simulink model "moto_linearization"  (R2026a)
settings: Solver=VariableStepAuto  StopTime=30
values from neighbouring files (symbols this model uses):
  ft = bs.FrontTire    [bikeSimToMotoParameters.m]
  Gf = Nsh.'*(Oh - B)    [bikeSimToMotoParameters.m]
  Ib = sum(I,3)    [bikeSimToMotoParameters.m]
  If = sum(I,3)    [bikeSimToMotoParameters.m]
  Ift = zeros(3)    [bikeSimToMotoParameters.m]
  Irt = zeros(3)    [bikeSimToMotoParameters.m]
  m = front_bodies(k).m    [bikeSimToMotoParameters.m]
  N = eye(3)    [bikeSimToMotoParameters.m]
  Ob = sum([rear_bodies.O].*[rear_bodies.m],2)/p.mb    [bikeSimToMotoParameters.m]
  p = motoParameters    [bikeSimToMotoParameters.m]    (also in moto_init.m = bikeSimToPrydeV2Parameters(bs,130/3.6); moto_trim_test.m = P{idx_vx}; steadyTurningTrimEqns.m = in3(41,:); steadyTurningTrimJac.m = in3(41,:))
  pf = fpacejka(bs.FrontTire.Pacejka)    [moto_trim_test.m]
  pr = fpacejka(bs.RearTire.Pacejka)    [moto_trim_test.m]
  rt = bs.RearTire    [bikeSimToMotoParameters.m]
  s = linspace(-pi,pi,36)'    [moto_init.m]
  sm = bs.SprungMass    [bikeSimToMotoParameters.m]
  X = zeros(ns,ns,12)    [moto_trim_test.m]
undefined symbols (not defined in the file or in its folder): mb, mh, Rr, Vlow, Y, Z
libraries: sm_lib x60, nesl_utility x51
(part 3 of 5)

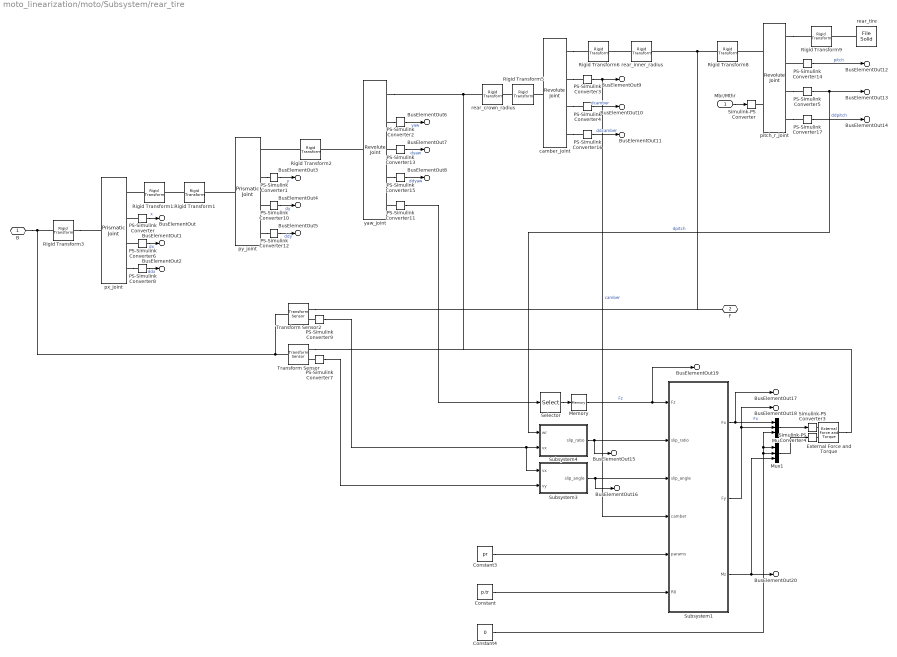
== system moto_linearization/moto/Subsystem/rear_tire ==
  Mbr/Mthr : Inport
  Constant : Constant  Value=p.tr
  Constant3 : Constant  Value=pr
  Constant4 : Constant  Value=0
  External Force and Torque : sm_lib/Forces and Torques/External Force and Torque  EnableForceX=off  EnableForceY=off  EnableForceZ=off  EnableForce=on  ForceResolutionFrame=AttachedFrame  EnableTorqueX=off  EnableTorqueY=off  EnableTorqueZ=off  EnableTorque=on  TorqueResolutionFrame=AttachedFrame
  Memory : Memory  InitialCondition=p.fzr  LinearizeAsDelay=on
  Mux : Mux  Inputs=3
  Mux1 : Mux  Inputs=3
  PS-Simulink Converter{,1..17} (18 alike) : nesl_utility/PS-Simulink Converter  PhysicalDomain=network_engine_domain  SubClassName=ps_output  LeftPortType=input  RightPortType=output  PseudoPeriodic=off  Frequencies=[]  VectorFormat=inherit  Unit=inherit  AffineConversion=off
  Rigid Transform1 : sm_lib/Frames and Transforms/Rigid Transform  RotationMethod=StandardAxis  FollAlignAxisA=+X  BaseAlignAxisA=+Y  FollAlignAxisB=+Y  BaseAlignAxisB=+Z  RotationStandardAxis=-X  RotationAngle=90  RotationAngleUnits=deg  RotationArbitraryAxis=[0 0 1]  RotationSequenceAxes=FollowerAxes  RotationSequence=XYX  RotationSequenceAngles=[0 0 0]  RotationSequenceAnglesUnits=deg  RotationMatrix=[1 0 0;0 1 0;0 0 1]  Quaternion=[1 0 0 0]  TranslationMethod=None  TranslationCartesianOffset=[0 0 0]  TranslationCartesianOffsetUnits=m  TranslationStandardAxis=+Z  TranslationStandardOffset=0  TranslationStandardOffsetUnits=m  TranslationROffset=0  TranslationROffsetUnits=m  TranslationThetaOffset=0  TranslationThetaOffsetUnits=deg  TranslationZOffset=0  TranslationZOffsetUnits=m
  Rigid Transform12 : sm_lib/Frames and Transforms/Rigid Transform  RotationMethod=StandardAxis  FollAlignAxisA=+X  BaseAlignAxisA=+Y  FollAlignAxisB=+Y  BaseAlignAxisB=+Z  RotationStandardAxis=-Y  RotationAngle=90  RotationAngleUnits=deg  RotationArbitraryAxis=[0 0 1]  RotationSequenceAxes=FollowerAxes  RotationSequence=XYX  RotationSequenceAngles=[0 0 0]  RotationSequenceAnglesUnits=deg  RotationMatrix=[1 0 0;0 1 0;0 0 1]  Quaternion=[1 0 0 0]  TranslationMethod=None  TranslationCartesianOffset=[0 0 0]  TranslationCartesianOffsetUnits=m  TranslationStandardAxis=+Z  TranslationStandardOffset=0  TranslationStandardOffsetUnits=m  TranslationROffset=0  TranslationROffsetUnits=m  TranslationThetaOffset=0  TranslationThetaOffsetUnits=deg  TranslationZOffset=0  TranslationZOffsetUnits=m
  Rigid Transform2 : sm_lib/Frames and Transforms/Rigid Transform  RotationMethod=StandardAxis  FollAlignAxisA=+X  BaseAlignAxisA=+Y  FollAlignAxisB=+Y  BaseAlignAxisB=+Z  RotationStandardAxis=+X  RotationAngle=90  RotationAngleUnits=deg  RotationArbitraryAxis=[0 0 1]  RotationSequenceAxes=FollowerAxes  RotationSequence=XYX  RotationSequenceAngles=[0 0 0]  RotationSequenceAnglesUnits=deg  RotationMatrix=[1 0 0;0 1 0;0 0 1]  Quaternion=[1 0 0 0]  TranslationMethod=None  TranslationCartesianOffset=[0 0 0]  TranslationCartesianOffsetUnits=m  TranslationStandardAxis=+Z  TranslationStandardOffset=0  TranslationStandardOffsetUnits=m  TranslationROffset=0  TranslationROffsetUnits=m  TranslationThetaOffset=0  TranslationThetaOffsetUnits=deg  TranslationZOffset=0  TranslationZOffsetUnits=m
  Rigid Transform3 : sm_lib/Frames and Transforms/Rigid Transform  RotationMethod=StandardAxis  FollAlignAxisA=+X  BaseAlignAxisA=+Y  FollAlignAxisB=+Y  BaseAlignAxisB=+Z  RotationStandardAxis=+Y  RotationAngle=90  RotationAngleUnits=deg  RotationArbitraryAxis=[0 0 1]  RotationSequenceAxes=FollowerAxes  RotationSequence=XYX  RotationSequenceAngles=[0 0 0]  RotationSequenceAnglesUnits=deg  RotationMatrix=[1 0 0;0 1 0;0 0 1]  Quaternion=[1 0 0 0]  TranslationMethod=None  TranslationCartesianOffset=[0 0 0]  TranslationCartesianOffsetUnits=m  TranslationStandardAxis=+Z  TranslationStandardOffset=0  TranslationStandardOffsetUnits=m  TranslationROffset=0  TranslationROffsetUnits=m  TranslationThetaOffset=0  TranslationThetaOffsetUnits=deg  TranslationZOffset=0  TranslationZOffsetUnits=m
  Rigid Transform5 : sm_lib/Frames and Transforms/Rigid Transform  RotationMethod=StandardAxis  FollAlignAxisA=+X  BaseAlignAxisA=+Y  FollAlignAxisB=+Y  BaseAlignAxisB=+Z  RotationStandardAxis=+Y  RotationAngle=90  RotationAngleUnits=deg  RotationArbitraryAxis=[0 0 1]  RotationSequenceAxes=FollowerAxes  RotationSequence=XYX  RotationSequenceAngles=[0 0 0]  RotationSequenceAnglesUnits=deg  RotationMatrix=[1 0 0;0 1 0;0 0 1]  Quaternion=[1 0 0 0]  TranslationMethod=None  TranslationCartesianOffset=[0 0 0]  TranslationCartesianOffsetUnits=m  TranslationStandardAxis=+Z  TranslationStandardOffset=0  TranslationStandardOffsetUnits=m  TranslationROffset=0  TranslationROffsetUnits=m  TranslationThetaOffset=0  TranslationThetaOffsetUnits=deg  TranslationZOffset=0  TranslationZOffsetUnits=m
  Rigid Transform6 : sm_lib/Frames and Transforms/Rigid Transform  RotationMethod=StandardAxis  FollAlignAxisA=+X  BaseAlignAxisA=+Y  FollAlignAxisB=+Y  BaseAlignAxisB=+Z  RotationStandardAxis=-Y  RotationAngle=90  RotationAngleUnits=deg  RotationArbitraryAxis=[0 0 1]  RotationSequenceAxes=FollowerAxes  RotationSequence=XYX  RotationSequenceAngles=[0 0 0]  RotationSequenceAnglesUnits=deg  RotationMatrix=[1 0 0;0 1 0;0 0 1]  Quaternion=[1 0 0 0]  TranslationMethod=None  TranslationCartesianOffset=[0 0 0]  TranslationCartesianOffsetUnits=m  TranslationStandardAxis=+Z  TranslationStandardOffset=0  TranslationStandardOffsetUnits=m  TranslationROffset=0  TranslationROffsetUnits=m  TranslationThetaOffset=0  TranslationThetaOffsetUnits=deg  TranslationZOffset=0  TranslationZOffsetUnits=m
  Rigid Transform8 : sm_lib/Frames and Transforms/Rigid Transform  RotationMethod=StandardAxis  FollAlignAxisA=+X  BaseAlignAxisA=+Y  FollAlignAxisB=+Y  BaseAlignAxisB=+Z  RotationStandardAxis=-X  RotationAngle=90  RotationAngleUnits=deg  RotationArbitraryAxis=[0 0 1]  RotationSequenceAxes=FollowerAxes  RotationSequence=XYX  RotationSequenceAngles=[0 0 0]  RotationSequenceAnglesUnits=deg  RotationMatrix=[1 0 0;0 1 0;0 0 1]  Quaternion=[1 0 0 0]  TranslationMethod=None  TranslationCartesianOffset=[0 0 0]  TranslationCartesianOffsetUnits=m  TranslationStandardAxis=+Z  TranslationStandardOffset=0  TranslationStandardOffsetUnits=m  TranslationROffset=0  TranslationROffsetUnits=m  TranslationThetaOffset=0  TranslationThetaOffsetUnits=deg  TranslationZOffset=0  TranslationZOffsetUnits=m
  Rigid Transform9 : sm_lib/Frames and Transforms/Rigid Transform  RotationMethod=StandardAxis  FollAlignAxisA=+X  BaseAlignAxisA=+Y  FollAlignAxisB=+Y  BaseAlignAxisB=+Z  RotationStandardAxis=+X  RotationAngle=90  RotationAngleUnits=deg  RotationArbitraryAxis=[0 0 1]  RotationSequenceAxes=FollowerAxes  RotationSequence=XYX  RotationSequenceAngles=[0 0 0]  RotationSequenceAnglesUnits=deg  RotationMatrix=[1 0 0;0 1 0;0 0 1]  Quaternion=[1 0 0 0]  TranslationMethod=None  TranslationCartesianOffset=[0 0 0]  TranslationCartesianOffsetUnits=m  TranslationStandardAxis=+Z  TranslationStandardOffset=0  TranslationStandardOffsetUnits=m  TranslationROffset=0  TranslationROffsetUnits=m  TranslationThetaOffset=0  TranslationThetaOffsetUnits=deg  TranslationZOffset=0  TranslationZOffsetUnits=m
  Selector : Selector  InputPortWidth=3  IndexOptions=Index vector (dialog)  Indices=3  OutputSizes=1
  Simulink-PS Converter : nesl_utility/Simulink-PS Converter  PhysicalDomain=network_engine_domain  SubClassName=ps_input  LeftPortType=input  RightPortType=output  PseudoPeriodic=off  Frequencies=[]  NoiseDistribution=none  NoiseParameters=[]  Unit=N*m  AffineConversion=off  FilteringAndDerivatives=provide  SimscapeFilterOrder=1  InputFilterTimeConstant=0.001  UdotUserProvided=0
  Simulink-PS Converter3 : nesl_utility/Simulink-PS Converter  PhysicalDomain=network_engine_domain  SubClassName=ps_input  LeftPortType=input  RightPortType=output  PseudoPeriodic=off  Frequencies=[]  NoiseDistribution=none  NoiseParameters=[]  Unit=N  AffineConversion=off  FilteringAndDerivatives=provide  SimscapeFilterOrder=1  InputFilterTimeConstant=0.001  UdotUserProvided=0
  Simulink-PS Converter4 : nesl_utility/Simulink-PS Converter  PhysicalDomain=network_engine_domain  SubClassName=ps_input  LeftPortType=input  RightPortType=output  PseudoPeriodic=off  Frequencies=[]  NoiseDistribution=none  NoiseParameters=[]  Unit=N*m  AffineConversion=off  FilteringAndDerivatives=provide  SimscapeFilterOrder=1  InputFilterTimeConstant=0.001  UdotUserProvided=0
  Subsystem1 : Subsystem
  Subsystem3 : Subsystem
  Subsystem4 : Subsystem
  Transform Sensor : sm_lib/Frames and Transforms/Transform Sensor  MeasurementFrame=NonRotatingFollower  RotationSequence=ZXY  SenseAngle=off  SenseAxis=off  SenseQ=off  SenseR=off  SenseRotationSequence=off  SenseOmegaX=off  SenseOmegaY=off  SenseOmegaZ=off  SenseOmega=off  SenseQDot=off  SenseRDot=off  SenseRotationSequenceDot=off  SenseAlphaX=off  SenseAlphaY=off  SenseAlphaZ=off  SenseAlpha=off  SenseQDDot=off  SenseRDDot=off  SenseX=off  SenseY=off  SenseZ=off  SenseXYZ=off  SenseRad=off  SenseAzim=off  SenseDist=off  SenseInc=off  SenseXDot=off  SenseYDot=on  SenseZDot=off  SenseXYZDot=off  SenseRadDot=off  SenseAzimDot=off  SenseDistDot=off  SenseIncDot=off  SenseXDDot=off  SenseYDDot=off  SenseZDDot=off  SenseXYZDDot=off  SenseRadDDot=off  SenseAzimDDot=off  SenseDistDDot=off  SenseIncDDot=off
  Transform Sensor2 : sm_lib/Frames and Transforms/Transform Sensor  MeasurementFrame=NonRotatingFollower  RotationSequence=ZXY  SenseAngle=off  SenseAxis=off  SenseQ=off  SenseR=off  SenseRotationSequence=off  SenseOmegaX=off  SenseOmegaY=off  SenseOmegaZ=off  SenseOmega=off  SenseQDot=off  SenseRDot=off  SenseRotationSequenceDot=off  SenseAlphaX=off  SenseAlphaY=off  SenseAlphaZ=off  SenseAlpha=off  SenseQDDot=off  SenseRDDot=off  SenseX=off  SenseY=off  SenseZ=off  SenseXYZ=off  SenseRad=off  SenseAzim=off  SenseDist=off  SenseInc=off  SenseXDot=on  SenseYDot=off  SenseZDot=off  SenseXYZDot=off  SenseRadDot=off  SenseAzimDot=off  SenseDistDot=off  SenseIncDot=off  SenseXDDot=off  SenseYDDot=off  SenseZDDot=off  SenseXYZDDot=off  SenseRadDDot=off  SenseAzimDDot=off  SenseDistDDot=off  SenseIncDDot=off
  camber_joint : sm_lib/Joints/Revolute Joint  JointMode=Normal  CompositeWrenchDir=FollowerOnBase  CompositeWrenchFrame=BaseFrame  SenseConstraintForce=off  SenseConstraintTorque=off  SenseTotalForce=off  SenseTotalTorque=off  PositionTargetSpecify=off  PositionTargetPriority=High  PositionTargetValue=0  PositionTargetValueUnits=deg  VelocityTargetSpecify=off  VelocityTargetPriority=High  VelocityTargetValue=0  VelocityTargetValueUnits=deg/s  EquilibriumPosition=0  EquilibriumPositionUnits=deg  SpringStiffness=0  SpringStiffnessUnits=N*m/deg  DampingCoefficient=0  DampingCoefficientUnits=N*m/(deg/s)  LowerLimitSpecify=off  LowerLimitBound=-90  LowerLimitBoundUnits=deg  LowerLimitStiffness=1e4  LowerLimitStiffnessUnits=N*m/deg  LowerLimitDamping=10  LowerLimitDampingUnits=N*m/(deg/s)  LowerLimitTransitionRegionWidth=0.1  LowerLimitTransitionRegionWidthUnits=deg  UpperLimitSpecify=off  UpperLimitBound=90  UpperLimitBoundUnits=deg  UpperLimitStiffness=1e4  UpperLimitStiffnessUnits=N*m/deg  UpperLimitDamping=10  UpperLimitDampingUnits=N*m/(deg/s)  UpperLimitTransitionRegionWidth=0.1  UpperLimitTransitionRegionWidthUnits=deg  TorqueActuationMode=NoTorque  MotionActuationMode=ComputedMotion  SensePosition=on  SenseVelocity=on  SenseAcceleration=on  SenseTorqueForce=off  SenseLowerLimitTorqueForce=off  SenseUpperLimitTorqueForce=off
  pitch_r_joint : sm_lib/Joints/Revolute Joint  JointMode=Normal  CompositeWrenchDir=FollowerOnBase  CompositeWrenchFrame=BaseFrame  SenseConstraintForce=off  SenseConstraintTorque=off  SenseTotalForce=off  SenseTotalTorque=off  PositionTargetSpecify=off  PositionTargetPriority=High  PositionTargetValue=0  PositionTargetValueUnits=deg  VelocityTargetSpecify=on  VelocityTargetPriority=Low  VelocityTargetValue=wr0  VelocityTargetValueUnits=rad/s  EquilibriumPosition=0  EquilibriumPositionUnits=deg  SpringStiffness=0  SpringStiffnessUnits=N*m/deg  DampingCoefficient=0  DampingCoefficientUnits=N*m/(deg/s)  LowerLimitSpecify=off  LowerLimitBound=-90  LowerLimitBoundUnits=deg  LowerLimitStiffness=1e4  LowerLimitStiffnessUnits=N*m/deg  LowerLimitDamping=10  LowerLimitDampingUnits=N*m/(deg/s)  LowerLimitTransitionRegionWidth=0.1  LowerLimitTransitionRegionWidthUnits=deg  UpperLimitSpecify=off  UpperLimitBound=90  UpperLimitBoundUnits=deg  UpperLimitStiffness=1e4  UpperLimitStiffnessUnits=N*m/deg  UpperLimitDamping=10  UpperLimitDampingUnits=N*m/(deg/s)  UpperLimitTransitionRegionWidth=0.1  UpperLimitTransitionRegionWidthUnits=deg  TorqueActuationMode=InputTorque  MotionActuationMode=ComputedMotion  SensePosition=on  SenseVelocity=on  SenseAcceleration=on  SenseTorqueForce=off  SenseLowerLimitTorqueForce=off  SenseUpperLimitTorqueForce=off
  px_joint : sm_lib/Joints/Prismatic Joint  JointMode=Normal  CompositeWrenchDir=FollowerOnBase  CompositeWrenchFrame=BaseFrame  SenseConstraintForce=off  SenseConstraintTorque=off  SenseTotalForce=off  SenseTotalTorque=off  PositionTargetSpecify=off  PositionTargetPriority=High  PositionTargetValue=0  PositionTargetValueUnits=m  VelocityTargetSpecify=on  VelocityTargetPriority=High  VelocityTargetValue=vx  VelocityTargetValueUnits=m/s  EquilibriumPosition=0  EquilibriumPositionUnits=m  SpringStiffness=0  SpringStiffnessUnits=N/m  DampingCoefficient=0  DampingCoefficientUnits=N/(m/s)  LowerLimitSpecify=off  LowerLimitBound=-1  LowerLimitBoundUnits=m  LowerLimitStiffness=1e6  LowerLimitStiffnessUnits=N/m  LowerLimitDamping=1e3  LowerLimitDampingUnits=N/(m/s)  LowerLimitTransitionRegionWidth=1e-4  LowerLimitTransitionRegionWidthUnits=m  UpperLimitSpecify=off  UpperLimitBound=1  UpperLimitBoundUnits=m  UpperLimitStiffness=1e6  UpperLimitStiffnessUnits=N/m  UpperLimitDamping=1e3  UpperLimitDampingUnits=N/(m/s)  UpperLimitTransitionRegionWidth=1e-4  UpperLimitTransitionRegionWidthUnits=m  TorqueActuationMode=NoTorque  MotionActuationMode=ComputedMotion  SensePosition=on  SenseVelocity=on  SenseAcceleration=on  SenseTorqueForce=off  SenseLowerLimitTorqueForce=off  SenseUpperLimitTorqueForce=off
  py_joint : sm_lib/Joints/Prismatic Joint  JointMode=Normal  CompositeWrenchDir=FollowerOnBase  CompositeWrenchFrame=BaseFrame  SenseConstraintForce=off  SenseConstraintTorque=off  SenseTotalForce=off  SenseTotalTorque=off  PositionTargetSpecify=off  PositionTargetPriority=High  PositionTargetValue=0  PositionTargetValueUnits=m  VelocityTargetSpecify=off  VelocityTargetPriority=High  VelocityTargetValue=0  VelocityTargetValueUnits=m/s  EquilibriumPosition=0  EquilibriumPositionUnits=m  SpringStiffness=0  SpringStiffnessUnits=N/m  DampingCoefficient=0  DampingCoefficientUnits=N/(m/s)  LowerLimitSpecify=off  LowerLimitBound=-1  LowerLimitBoundUnits=m  LowerLimitStiffness=1e6  LowerLimitStiffnessUnits=N/m  LowerLimitDamping=1e3  LowerLimitDampingUnits=N/(m/s)  LowerLimitTransitionRegionWidth=1e-4  LowerLimitTransitionRegionWidthUnits=m  UpperLimitSpecify=off  UpperLimitBound=1  UpperLimitBoundUnits=m  UpperLimitStiffness=1e6  UpperLimitStiffnessUnits=N/m  UpperLimitDamping=1e3  UpperLimitDampingUnits=N/(m/s)  UpperLimitTransitionRegionWidth=1e-4  UpperLimitTransitionRegionWidthUnits=m  TorqueActuationMode=NoTorque  MotionActuationMode=ComputedMotion  SensePosition=on  SenseVelocity=on  SenseAcceleration=on  SenseTorqueForce=off  SenseLowerLimitTorqueForce=off  SenseUpperLimitTorqueForce=off
  rear_crown_radius : sm_lib/Frames and Transforms/Rigid Transform  RotationMethod=StandardAxis  FollAlignAxisA=+X  BaseAlignAxisA=+Y  FollAlignAxisB=+Y  BaseAlignAxisB=+Z  RotationStandardAxis=+Z  RotationAngle=0  RotationAngleUnits=deg  RotationArbitraryAxis=[0 0 1]  RotationSequenceAxes=FollowerAxes  RotationSequence=XYX  RotationSequenceAngles=[0 0 0]  RotationSequenceAnglesUnits=deg  RotationMatrix=[1 0 0;0 1 0;0 0 1]  Quaternion=[1 0 0 0]  TranslationMethod=StandardAxis  TranslationCartesianOffset=[0 0 0]  TranslationCartesianOffsetUnits=m  TranslationStandardAxis=+Z  TranslationStandardOffset=p.tr  TranslationStandardOffsetUnits=m  TranslationROffset=0  TranslationROffsetUnits=m  TranslationThetaOffset=0  TranslationThetaOffsetUnits=deg  TranslationZOffset=0  TranslationZOffsetUnits=m
  rear_inner_radius : sm_lib/Frames and Transforms/Rigid Transform  RotationMethod=StandardAxis  FollAlignAxisA=+X  BaseAlignAxisA=+Y  FollAlignAxisB=+Y  BaseAlignAxisB=+Z  RotationStandardAxis=+Z  RotationAngle=0  RotationAngleUnits=deg  RotationArbitraryAxis=[0 0 1]  RotationSequenceAxes=FollowerAxes  RotationSequence=XYX  RotationSequenceAngles=[0 0 0]  RotationSequenceAnglesUnits=deg  RotationMatrix=[1 0 0;0 1 0;0 0 1]  Quaternion=[1 0 0 0]  TranslationMethod=StandardAxis  TranslationCartesianOffset=[0 0 0]  TranslationCartesianOffsetUnits=m  TranslationStandardAxis=+Z  TranslationStandardOffset=p.rr  TranslationStandardOffsetUnits=m  TranslationROffset=0  TranslationROffsetUnits=m  TranslationThetaOffset=0  TranslationThetaOffsetUnits=deg  TranslationZOffset=0  TranslationZOffsetUnits=m
  rear_tire : sm_lib/Body Elements/File Solid  ExtGeomFileName=rear_tire.stl  UnitType=Custom  ExtGeomFileUnits=mm  StepReaderType=HEX  ExportConvexHullGeometry=off  InertiaType=Custom  BasedOnType=DensityFromFile  Density=1000  DensityUnits=kg/m^3  Mass=rt.Mass  MassUnits=kg  CenterOfMass=[0 0 0]  CenterOfMassUnits=m  MomentsOfInertia=diag(Irt)  MomentsOfInertiaUnits=kg*m^2  ProductsOfInertia=[0 0 0]  ProductsOfInertiaUnits=kg*m^2  GraphicType=FromGeometry  MarkerShape=Sphere  MarkerSize=10  GraphicVisPropType=SimpleVisualProperties  GraphicDiffuseColor=[0.5 0.5 0.5]  GraphicOpacity=1  GraphicSpecularColor=[0.5 0.5 0.5 1.0]  GraphicAmbientColor=[0.15 0.15 0.15 1.0]  GraphicEmissiveColor=[0.0 0.0 0.0 1.0]  GraphicShininess=75  DoExposeReferenceFrame=on  SerializedFrames=<Frames/>
  yaw_joint : sm_lib/Joints/Revolute Joint  JointMode=Normal  CompositeWrenchDir=BaseOnFollower  CompositeWrenchFrame=FollowerFrame  SenseConstraintForce=on  SenseConstraintTorque=off  SenseTotalForce=off  SenseTotalTorque=off  PositionTargetSpecify=off  PositionTargetPriority=High  PositionTargetValue=0  PositionTargetValueUnits=deg  VelocityTargetSpecify=off  VelocityTargetPriority=High  VelocityTargetValue=0  VelocityTargetValueUnits=deg/s  EquilibriumPosition=0  EquilibriumPositionUnits=deg  SpringStiffness=0  SpringStiffnessUnits=N*m/deg  DampingCoefficient=0  DampingCoefficientUnits=N*m/(deg/s)  LowerLimitSpecify=off  LowerLimitBound=-90  LowerLimitBoundUnits=deg  LowerLimitStiffness=1e4  LowerLimitStiffnessUnits=N*m/deg  LowerLimitDamping=10  LowerLimitDampingUnits=N*m/(deg/s)  LowerLimitTransitionRegionWidth=0.1  LowerLimitTransitionRegionWidthUnits=deg  UpperLimitSpecify=off  UpperLimitBound=90  UpperLimitBoundUnits=deg  UpperLimitStiffness=1e4  UpperLimitStiffnessUnits=N*m/deg  UpperLimitDamping=10  UpperLimitDampingUnits=N*m/(deg/s)  UpperLimitTransitionRegionWidth=0.1  UpperLimitTransitionRegionWidthUnits=deg  TorqueActuationMode=NoTorque  MotionActuationMode=ComputedMotion  SensePosition=on  SenseVelocity=on  SenseAcceleration=on  SenseTorqueForce=off  SenseLowerLimitTorqueForce=off  SenseUpperLimitTorqueForce=off
  B : PMIOPort  Side=Left
  F : PMIOPort  Port=2  Side=Right
  BusElementOut : Outport  PortName=RearTire  Element=Position.X
  BusElementOut3 : Outport  PortName=RearTire  Element=Position.Y
  BusElementOut6 : Outport  PortName=RearTire  Element=Position.Yaw
  BusElementOut9 : Outport  PortName=RearTire  Element=Position.Camber
  BusElementOut12 : Outport  PortName=RearTire  Element=Position.Pitch
  BusElementOut1 : Outport  PortName=RearTire  Element=Velocity.X
  BusElementOut4 : Outport  PortName=RearTire  Element=Velocity.Y
  BusElementOut7 : Outport  PortName=RearTire  Element=Velocity.Yaw
  BusElementOut10 : Outport  PortName=RearTire  Element=Velocity.Camber
  BusElementOut13 : Outport  PortName=RearTire  Element=Velocity.Pitch
  BusElementOut2 : Outport  PortName=RearTire  Element=Acceleration.X
  BusElementOut5 : Outport  PortName=RearTire  Element=Acceleration.Y
  BusElementOut8 : Outport  PortName=RearTire  Element=Acceleration.Yaw
  BusElementOut11 : Outport  PortName=RearTire  Element=Acceleration.Camber
  BusElementOut14 : Outport  PortName=RearTire  Element=Acceleration.Pitch
  BusElementOut15 : Outport  PortName=RearTire  Element=Slip.Ratio
  BusElementOut16 : Outport  PortName=RearTire  Element=Slip.Angle
  BusElementOut17 : Outport  PortName=RearTire  Element=Wrench.Fx
  BusElementOut18 : Outport  PortName=RearTire  Element=Wrench.Fy
  BusElementOut19 : Outport  PortName=RearTire  Element=Wrench.Fz
  BusElementOut20 : Outport  PortName=RearTire  Element=Wrench.Mz
  wires:
  Mux1/1 -> Simulink-PS Converter4/1
  Mux/1 -> Simulink-PS Converter3/1
  Mbr/Mthr/1 -> Simulink-PS Converter/1
  PS-Simulink Converter/1 -> BusElementOut/1  "x"
  PS-Simulink Converter6/1 -> BusElementOut1/1  "dx"
  PS-Simulink Converter8/1 -> BusElementOut2/1  "ddx"
  PS-Simulink Converter1/1 -> BusElementOut3/1  "y"
  PS-Simulink Converter10/1 -> BusElementOut4/1  "dy"
  PS-Simulink Converter12/1 -> BusElementOut5/1  "ddy"
  PS-Simulink Converter2/1 -> BusElementOut6/1  "yaw"
  PS-Simulink Converter13/1 -> BusElementOut7/1  "dyaw"
  PS-Simulink Converter15/1 -> BusElementOut8/1  "ddyaw"
  PS-Simulink Converter3/1 -> BusElementOut9/1, Subsystem1/4(camber)  "camber"
  PS-Simulink Converter4/1 -> BusElementOut10/1  "dcamber"
  PS-Simulink Converter16/1 -> BusElementOut11/1  "ddcamber"
  PS-Simulink Converter14/1 -> BusElementOut12/1  "pitch"
  PS-Simulink Converter5/1 -> BusElementOut13/1, Subsystem4/1(wr)  "dpitch"
  PS-Simulink Converter17/1 -> BusElementOut14/1  "ddpitch"
  PS-Simulink Converter11/1 -> Selector/1
  PS-Simulink Converter7/1 -> Subsystem3/2(vy)
  Subsystem1/1(Fx) -> BusElementOut17/1, Mux/1  "Fx"
  Memory/1 -> BusElementOut19/1, Subsystem1/1(Fz)  "Fz"
  Selector/1 -> Memory/1
  Subsystem3/1(slip_angle) -> Subsystem1/3(slip_angle), BusElementOut16/1
  Constant4/1 -> Mux1/2, Mux/3, Mux1/1
  Constant3/1 -> Subsystem1/5(params)
  Subsystem4/1(slip_ratio) -> Subsystem1/2(slip_ratio), BusElementOut15/1
  Constant/1 -> Subsystem1/6(R0)
  Subsystem1/2(Fy) -> BusElementOut18/1, Mux/2
  Subsystem1/3(Mz) -> BusElementOut20/1, Mux1/3
  PS-Simulink Converter9/1 -> Subsystem3/1(vx), Subsystem4/2(vx)
  connections:
  yaw_joint/RConn2 -- PS-Simulink Converter2/LConn1
  yaw_joint/RConn1 -- Transform Sensor/RConn1 -- External Force and Torque/RConn1 -- rear_crown_radius/LConn1
  Rigid Transform1/LConn1 -- Rigid Transform12/RConn1
  camber_joint/RConn1 -- Rigid Transform6/LConn1
  Rigid Transform8/LConn1 -- F/RConn1 -- Transform Sensor2/RConn1 -- rear_inner_radius/RConn1
  py_joint/LConn1 -- Rigid Transform1/RConn1
  Rigid Transform3/RConn1 -- px_joint/LConn1
  rear_inner_radius/LConn1 -- Rigid Transform6/RConn1
  rear_tire/RConn1 -- Rigid Transform9/RConn1
  Simulink-PS Converter4/RConn1 -- External Force and Torque/LConn2
  PS-Simulink Converter/LConn1 -- px_joint/RConn2
  PS-Simulink Converter7/LConn1 -- Transform Sensor/RConn2
  Simulink-PS Converter/RConn1 -- pitch_r_joint/LConn2
  Rigid Transform12/LConn1 -- px_joint/RConn1
  Rigid Transform5/LConn1 -- rear_crown_radius/RConn1
  PS-Simulink Converter11/LConn1 -- yaw_joint/RConn5
  PS-Simulink Converter9/LConn1 -- Transform Sensor2/RConn2
  py_joint/RConn2 -- PS-Simulink Converter1/LConn1
  pitch_r_joint/LConn1 -- Rigid Transform8/RConn1
  Rigid Transform2/LConn1 -- py_joint/RConn1
  camber_joint/RConn2 -- PS-Simulink Converter3/LConn1
  External Force and Torque/LConn1 -- Simulink-PS Converter3/RConn1
  pitch_r_joint/RConn3 -- PS-Simulink Converter5/LConn1
  camber_joint/LConn1 -- Rigid Transform5/RConn1
  yaw_joint/LConn1 -- Rigid Transform2/RConn1
  pitch_r_joint/RConn1 -- Rigid Transform9/LConn1
  PS-Simulink Converter14/LConn1 -- pitch_r_joint/RConn2
  B/RConn1 -- Transform Sensor/LConn1 -- Transform Sensor2/LConn1 -- Rigid Transform3/LConn1
  camber_joint/RConn3 -- PS-Simulink Converter4/LConn1
  PS-Simulink Converter6/LConn1 -- px_joint/RConn3
  px_joint/RConn4 -- PS-Simulink Converter8/LConn1
  PS-Simulink Converter10/LConn1 -- py_joint/RConn3
  py_joint/RConn4 -- PS-Simulink Converter12/LConn1
  PS-Simulink Converter13/LConn1 -- yaw_joint/RConn3
  yaw_joint/RConn4 -- PS-Simulink Converter15/LConn1
  camber_joint/RConn4 -- PS-Simulink Converter16/LConn1
  pitch_r_joint/RConn4 -- PS-Simulink Converter17/LConn1

== system moto_linearization/moto/Subsystem/front_tire/Subsystem1 ==
  Fz : Inport
  slip_ratio : Inport  Port=2
  slip_angle : Inport  Port=3
  camber : Inport  Port=4
  params : Inport  Port=5
  R0 : Inport  Port=6
  Aligning moment (combined slip) : Subsystem
  Gain : Gain  Gain=0
  Horizontal shift : Subsystem
  Lateral force (combined slip) : Subsystem
  "Lateral force (combined slip, no camber)" : Subsystem
  Lateral force (pure slip) : Subsystem
  "Lateral force (pure slip, no camber)" : Subsystem
  Longitudinal force (combined slip) : Subsystem
  Longitudinal force (pure slip) : Subsystem
  MF bus : Subsystem
  Normalized normal force : Subsystem
  Residual slip : Subsystem
  Trail slip : Subsystem
  Fx : Outport
  Fy : Outport  Port=2
  Mz : Outport  Port=3
  wires:
  Fz/1 -> "Lateral force (pure slip, no camber)"/2(Fz), Aligning moment (combined slip)/2(Fz), Lateral force (pure slip)/2(Fz), Normalized normal force/1(Fz), Longitudinal force (pure slip)/1(Fz)  "Fz"
  Normalized normal force/1(dfz) -> "Lateral force (pure slip, no camber)"/1(dfz), Horizontal shift/1(dfz), Aligning moment (combined slip)/1(dfz), Lateral force (pure slip)/1(dfz), Longitudinal force (pure slip)/2(dfz)  "dfz"
  slip_ratio/1 -> Longitudinal force (pure slip)/3(slip_ratio), Longitudinal force (combined slip)/2(slip_ratio), "Lateral force (combined slip, no camber)"/2(slip_ratio), Trail slip/1(slip_ratio), Residual slip/1(slip_ratio), Lateral force (combined slip)/2(slip_ratio)  "slip_ratio"
  params/1 -> MF bus/1(params)  "params"
  MF bus/1(MF) -> Normalized normal force/2(MF), Longitudinal force (pure slip)/4(MF), "Lateral force (pure slip, no camber)"/5(MF), Horizontal shift/3(MF), Lateral force (pure slip)/5(MF), "Lateral force (combined slip, no camber)"/4(MF), Aligning moment (combined slip)/9(MF), Lateral force (combined slip)/4(MF), Longitudinal force (combined slip)/4(MF)  "MF"
  slip_angle/1 -> "Lateral force (pure slip, no camber)"/3(slip), "Lateral force (combined slip, no camber)"/3(slip_angle), Longitudinal force (combined slip)/3(slip_angle), Lateral force (combined slip)/3(slip_angle), Residual slip/2(slip_angle), Trail slip/2(slip_angle), Aligning moment (combined slip)/7(slip_angle), Lateral force (pure slip)/3(slip)  "slip_angle"
  camber/1 -> Horizontal shift/2(camber), Aligning moment (combined slip)/5(camber), Lateral force (pure slip)/4(camber), Gain/1  "camber"
  Longitudinal force (pure slip)/1(Info) -> Trail slip/3(Longitudinal), Residual slip/4(Longitudinal)
  "Lateral force (pure slip, no camber)"/1(Info) -> Trail slip/4(Lateral), Residual slip/5(Lateral)
  Longitudinal force (pure slip)/2(Fx0) -> Longitudinal force (combined slip)/1(Fx0)  "Fx0"
  Lateral force (pure slip)/2(Fy0) -> Lateral force (combined slip)/1(Fy0)
  Gain/1 -> "Lateral force (pure slip, no camber)"/4(camber)
  "Lateral force (pure slip, no camber)"/2(Fy0) -> "Lateral force (combined slip, no camber)"/1(Fy0)
  Horizontal shift/1(SHr) -> Residual slip/3(SHr)
  Residual slip/1(residual_slip) -> Aligning moment (combined slip)/3(residual_slip)
  Trail slip/1(trail_slip) -> Aligning moment (combined slip)/4(trail_slip)
  "Lateral force (combined slip, no camber)"/1(Fy) -> Aligning moment (combined slip)/6(Fyg0)
  Lateral force (pure slip)/1(Info) -> Aligning moment (combined slip)/8(Lateral)
  Longitudinal force (combined slip)/1(Fx) -> Fx/1
  Lateral force (combined slip)/1(Fy) -> Fy/1
  Aligning moment (combined slip)/1(Mz) -> Mz/1
  R0/1 -> Aligning moment (combined slip)/10(R0)

== system moto_linearization/moto/Subsystem/front_tire/Subsystem3 ==
  vx : Inport
  vy : Inport  Port=2
  Abs : Abs  SaturateOnIntegerOverflow=off
  Atan : Trigonometry  Operator=atan
  Constant : Constant  Value=p.rlry
  Constant1 : Constant
  Constant2 : Constant  Value=Vlow
  Divide : Product  Inputs=*/
  Divide1 : Product  Inputs=*/
  Gain : Gain  Gain=0.9
  Integrator : Integrator
  Product : Product
  Product1 : Product
  Sum : Sum  Inputs=|-+
  Sum1 : Sum  Inputs=-+|
  Sum2 : Sum  Inputs=|-+
  Switch : Switch  Criteria=u2 > Threshold  Threshold=Vlow  SaturateOnIntegerOverflow=off  InputSameDT=off
  slip_angle : Outport
  wires:
  Product/1 -> Sum/1
  Sum/1 -> Divide/1
  Divide/1 -> Integrator/1
  Constant2/1 -> Divide1/2, Sum1/2
  Constant/1 -> Switch/1, Product1/1
  Switch/1 -> Divide/2
  Product1/1 -> Switch/3
  Integrator/1 -> Product/2, Atan/1
  vx/1 -> Abs/1
  vy/1 -> Sum/2
  Abs/1 -> Product/1, Switch/2, Sum1/1
  Sum1/1 -> Gain/1
  Gain/1 -> Divide1/1
  Divide1/1 -> Sum2/1
  Constant1/1 -> Sum2/2
  Sum2/1 -> Product1/2
  Atan/1 -> slip_angle/1

== system moto_linearization/moto/Subsystem/front_tire/Subsystem4 ==
  wr : Inport
  vx : Inport  Port=2
  Abs : Abs  SaturateOnIntegerOverflow=off
  Abs1 : Abs  Commented=on  SaturateOnIntegerOverflow=off
  Constant : Constant
  Constant1 : Constant  Commented=on
  Divide : Product  Commented=on  Inputs=*/
  Gain : Gain  Gain=p.Rr
  Gain1 : Gain  Gain=1/p.rlrx
  Gain2 : Gain  Commented=on  Gain=1/Rr
  Integrator : Integrator
  Product : Product
  Product1 : Product
  Sign : Signum
  Sum : Sum  Inputs=|+-
  Sum1 : Sum  Inputs=|++
  Sum2 : Sum  Commented=on  Inputs=|+-
  slip_ratio : Outport
  wires:
  ? -> Gain2/1
  Gain2/1 -> Abs1/1
  ? -> Divide/1
  Abs1/1 -> Divide/2
  Divide/1 -> Sum2/1
  Constant1/1 -> Sum2/2
  Sum2/1 -> ?
  wr/1 -> Product/1
  Sign/1 -> Product/2
  vx/1 -> Abs/1, Sign/1
  Product/1 -> Gain/1
  Gain/1 -> Sum/1
  Abs/1 -> Product1/1
  Product1/1 -> Sum/2
  Sum1/1 -> Product1/2
  Constant/1 -> Sum1/1
  Sum/1 -> Gain1/1
  Gain1/1 -> Integrator/1
  Integrator/1 -> slip_ratio/1, Sum1/2

== system moto_linearization/moto/Subsystem/rear_tire/Subsystem1 ==
  Fz : Inport
  slip_ratio : Inport  Port=2
  slip_angle : Inport  Port=3
  camber : Inport  Port=4
  params : Inport  Port=5
  R0 : Inport  Port=6
  Aligning moment (combined slip) : Subsystem
  Gain : Gain  Gain=0
  Horizontal shift : Subsystem
  Lateral force (combined slip) : Subsystem
  "Lateral force (combined slip, no camber)" : Subsystem
  Lateral force (pure slip) : Subsystem
  "Lateral force (pure slip, no camber)" : Subsystem
  Longitudinal force (combined slip) : Subsystem
  Longitudinal force (pure slip) : Subsystem
  MF bus : Subsystem
  Normalized normal force : Subsystem
  Residual slip : Subsystem
  Trail slip : Subsystem
  Fx : Outport
  Fy : Outport  Port=2
  Mz : Outport  Port=3
  wires:
  Fz/1 -> "Lateral force (pure slip, no camber)"/2(Fz), Aligning moment (combined slip)/2(Fz), Lateral force (pure slip)/2(Fz), Normalized normal force/1(Fz), Longitudinal force (pure slip)/1(Fz)  "Fz"
  Normalized normal force/1(dfz) -> "Lateral force (pure slip, no camber)"/1(dfz), Horizontal shift/1(dfz), Aligning moment (combined slip)/1(dfz), Lateral force (pure slip)/1(dfz), Longitudinal force (pure slip)/2(dfz)  "dfz"
  slip_ratio/1 -> Longitudinal force (pure slip)/3(slip_ratio), Longitudinal force (combined slip)/2(slip_ratio), "Lateral force (combined slip, no camber)"/2(slip_ratio), Trail slip/1(slip_ratio), Residual slip/1(slip_ratio), Lateral force (combined slip)/2(slip_ratio)  "slip_ratio"
  params/1 -> MF bus/1(params)  "params"
  MF bus/1(MF) -> Normalized normal force/2(MF), Longitudinal force (pure slip)/4(MF), "Lateral force (pure slip, no camber)"/5(MF), Horizontal shift/3(MF), Lateral force (pure slip)/5(MF), "Lateral force (combined slip, no camber)"/4(MF), Aligning moment (combined slip)/9(MF), Lateral force (combined slip)/4(MF), Longitudinal force (combined slip)/4(MF)  "MF"
  slip_angle/1 -> "Lateral force (pure slip, no camber)"/3(slip), "Lateral force (combined slip, no camber)"/3(slip_angle), Longitudinal force (combined slip)/3(slip_angle), Lateral force (combined slip)/3(slip_angle), Residual slip/2(slip_angle), Trail slip/2(slip_angle), Aligning moment (combined slip)/7(slip_angle), Lateral force (pure slip)/3(slip)  "slip_angle"
  camber/1 -> Horizontal shift/2(camber), Aligning moment (combined slip)/5(camber), Lateral force (pure slip)/4(camber), Gain/1  "camber"
  Longitudinal force (pure slip)/1(Info) -> Trail slip/3(Longitudinal), Residual slip/4(Longitudinal)
  "Lateral force (pure slip, no camber)"/1(Info) -> Trail slip/4(Lateral), Residual slip/5(Lateral)
  Longitudinal force (pure slip)/2(Fx0) -> Longitudinal force (combined slip)/1(Fx0)  "Fx0"
  Lateral force (pure slip)/2(Fy0) -> Lateral force (combined slip)/1(Fy0)
  Gain/1 -> "Lateral force (pure slip, no camber)"/4(camber)
  "Lateral force (pure slip, no camber)"/2(Fy0) -> "Lateral force (combined slip, no camber)"/1(Fy0)
  Horizontal shift/1(SHr) -> Residual slip/3(SHr)
  Residual slip/1(residual_slip) -> Aligning moment (combined slip)/3(residual_slip)
  Trail slip/1(trail_slip) -> Aligning moment (combined slip)/4(trail_slip)
  "Lateral force (combined slip, no camber)"/1(Fy) -> Aligning moment (combined slip)/6(Fyg0)
  Lateral force (pure slip)/1(Info) -> Aligning moment (combined slip)/8(Lateral)
  Longitudinal force (combined slip)/1(Fx) -> Fx/1
  Lateral force (combined slip)/1(Fy) -> Fy/1
  Aligning moment (combined slip)/1(Mz) -> Mz/1
  R0/1 -> Aligning moment (combined slip)/10(R0)

== system moto_linearization/moto/Subsystem/rear_tire/Subsystem3 ==
  vx : Inport
  vy : Inport  Port=2
  Abs : Abs  SaturateOnIntegerOverflow=off
  Atan : Trigonometry  Operator=atan
  Constant : Constant  Value=p.rlry
  Constant1 : Constant
  Constant2 : Constant  Value=Vlow
  Divide : Product  Inputs=*/
  Divide1 : Product  Inputs=*/
  Gain : Gain  Gain=0.9
  Integrator : Integrator
  Product : Product
  Product1 : Product
  Sum : Sum  Inputs=|-+
  Sum1 : Sum  Inputs=-+|
  Sum2 : Sum  Inputs=|-+
  Switch : Switch  Criteria=u2 > Threshold  Threshold=Vlow  SaturateOnIntegerOverflow=off  InputSameDT=off
  slip_angle : Outport
  wires:
  Product/1 -> Sum/1
  Sum/1 -> Divide/1
  Divide/1 -> Integrator/1
  Constant2/1 -> Divide1/2, Sum1/2
  Constant/1 -> Switch/1, Product1/1
  Switch/1 -> Divide/2
  Product1/1 -> Switch/3
  Integrator/1 -> Product/2, Atan/1
  vx/1 -> Abs/1
  vy/1 -> Sum/2
  Abs/1 -> Product/1, Switch/2, Sum1/1
  Sum1/1 -> Gain/1
  Gain/1 -> Divide1/1
  Divide1/1 -> Sum2/1
  Constant1/1 -> Sum2/2
  Sum2/1 -> Product1/2
  Atan/1 -> slip_angle/1

== system moto_linearization/moto/Subsystem/rear_tire/Subsystem4 ==
  wr : Inport
  vx : Inport  Port=2
  Abs : Abs  SaturateOnIntegerOverflow=off
  Abs1 : Abs  Commented=on  SaturateOnIntegerOverflow=off
  Constant : Constant
  Constant1 : Constant  Commented=on
  Divide : Product  Commented=on  Inputs=*/
  Gain : Gain  Gain=p.Rr
  Gain1 : Gain  Gain=1/p.rlrx
  Gain2 : Gain  Commented=on  Gain=1/Rr
  Integrator : Integrator
  Product : Product
  Product1 : Product
  Sign : Signum
  Sum : Sum  Inputs=|+-
  Sum1 : Sum  Inputs=|++
  Sum2 : Sum  Commented=on  Inputs=|+-
  slip_ratio : Outport
  wires:
  ? -> Gain2/1
  Gain2/1 -> Abs1/1
  ? -> Divide/1
  Abs1/1 -> Divide/2
  Divide/1 -> Sum2/1
  Constant1/1 -> Sum2/2
  Sum2/1 -> ?
  wr/1 -> Product/1
  Sign/1 -> Product/2
  vx/1 -> Abs/1, Sign/1
  Product/1 -> Gain/1
  Gain/1 -> Sum/1
  Abs/1 -> Product1/1
  Product1/1 -> Sum/2
  Sum1/1 -> Product1/2
  Constant/1 -> Sum1/1
  Sum/1 -> Gain1/1
  Gain1/1 -> Integrator/1
  Integrator/1 -> slip_ratio/1, Sum1/2

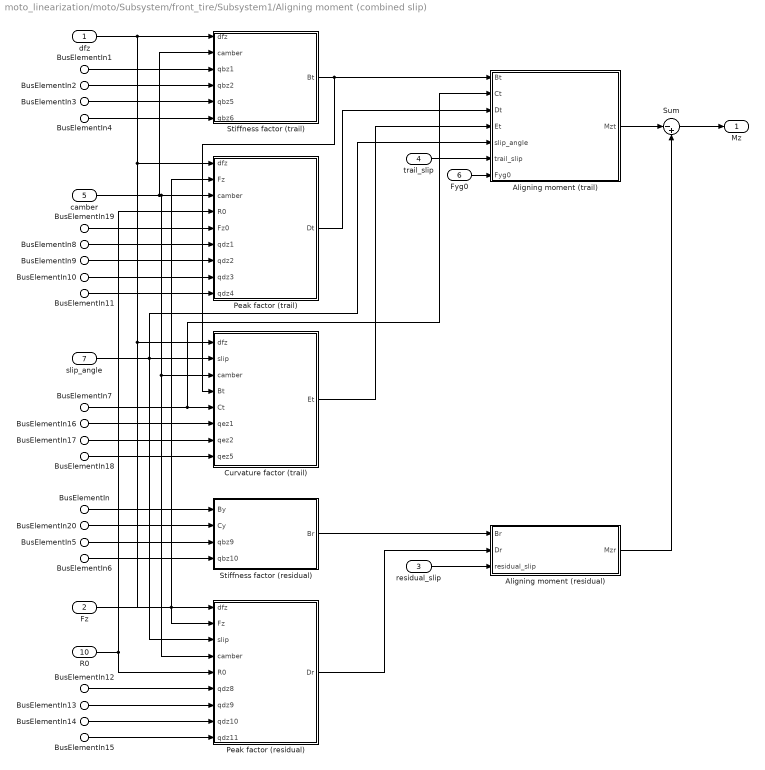
== system moto_linearization/moto/Subsystem/front_tire/Subsystem1/Aligning moment (combined slip) ==
  dfz : Inport
  Fz : Inport  Port=2
  residual_slip : Inport  Port=3
  trail_slip : Inport  Port=4
  camber : Inport  Port=5
  Fyg0 : Inport  Port=6
  slip_angle : Inport  Port=7
  BusElementIn : Inport  Port=8  PortName=Lateral  Element=By
  BusElementIn1 : Inport  Port=9  PortName=MF  Element=qbz1
  BusElementIn2 : Inport  Port=9  PortName=MF  Element=qbz2
  BusElementIn3 : Inport  Port=9  PortName=MF  Element=qbz5
  BusElementIn4 : Inport  Port=9  PortName=MF  Element=qbz6
  BusElementIn5 : Inport  Port=9  PortName=MF  Element=qbz9
  BusElementIn6 : Inport  Port=9  PortName=MF  Element=qbz10
  BusElementIn7 : Inport  Port=9  PortName=MF  Element=qcz1
  BusElementIn8 : Inport  Port=9  PortName=MF  Element=qdz1
  BusElementIn9 : Inport  Port=9  PortName=MF  Element=qdz2
  BusElementIn10 : Inport  Port=9  PortName=MF  Element=qdz3
  BusElementIn11 : Inport  Port=9  PortName=MF  Element=qdz4
  BusElementIn12 : Inport  Port=9  PortName=MF  Element=qdz8
  BusElementIn13 : Inport  Port=9  PortName=MF  Element=qdz9
  BusElementIn14 : Inport  Port=9  PortName=MF  Element=qdz10
  BusElementIn15 : Inport  Port=9  PortName=MF  Element=qdz11
  BusElementIn16 : Inport  Port=9  PortName=MF  Element=qez1
  BusElementIn17 : Inport  Port=9  PortName=MF  Element=qez2
  BusElementIn18 : Inport  Port=9  PortName=MF  Element=qez5
  BusElementIn19 : Inport  Port=9  PortName=MF  Element=fz0
  BusElementIn20 : Inport  Port=9  PortName=MF  Element=pcy1
  R0 : Inport  Port=10
  Aligning moment (residual) : Subsystem
  Aligning moment (trail) : Subsystem
  Curvature factor (trail) : Subsystem
  Peak factor (residual) : Subsystem
  Peak factor (trail) : Subsystem
  Stiffness factor (residual) : Subsystem
  Stiffness factor (trail) : Subsystem
  Sum : Sum  Inputs=|-+
  Mz : Outport
  wires:
  camber/1 -> Peak factor (residual)/4(camber), Curvature factor (trail)/3(camber), Peak factor (trail)/3(camber), Stiffness factor (trail)/2(camber)
  BusElementIn4/1 -> Stiffness factor (trail)/6(qbz6)
  Peak factor (residual)/1(Dr) -> Aligning moment (residual)/2(Dr)
  slip_angle/1 -> Curvature factor (trail)/2(slip), Aligning moment (trail)/5(slip_angle), Peak factor (residual)/3(slip)
  BusElementIn7/1 -> Aligning moment (trail)/2(Ct), Curvature factor (trail)/5(Ct)
  Aligning moment (residual)/1(Mzr) -> Sum/2
  BusElementIn5/1 -> Stiffness factor (residual)/3(qbz9)
  Aligning moment (trail)/1(Mzt) -> Sum/1
  dfz/1 -> Peak factor (residual)/1(dfz), Curvature factor (trail)/1(dfz), Peak factor (trail)/1(dfz), Stiffness factor (trail)/1(dfz)
  residual_slip/1 -> Aligning moment (residual)/3(residual_slip)
  BusElementIn16/1 -> Curvature factor (trail)/6(qez1)
  Stiffness factor (trail)/1(Bt) -> Aligning moment (trail)/1(Bt), Curvature factor (trail)/4(Bt)
  BusElementIn/1 -> Stiffness factor (residual)/1(By)
  Stiffness factor (residual)/1(Br) -> Aligning moment (residual)/1(Br)
  Fz/1 -> Peak factor (trail)/2(Fz), Peak factor (residual)/2(Fz)
  BusElementIn18/1 -> Curvature factor (trail)/8(qez5)
  R0/1 -> Peak factor (residual)/5(R0), Peak factor (trail)/4(R0)
  Curvature factor (trail)/1(Et) -> Aligning moment (trail)/4(Et)
  BusElementIn19/1 -> Peak factor (trail)/5(Fz0)
  Peak factor (trail)/1(Dt) -> Aligning moment (trail)/3(Dt)
  BusElementIn8/1 -> Peak factor (trail)/6(qdz1)
  BusElementIn14/1 -> Peak factor (residual)/8(qdz10)
  BusElementIn11/1 -> Peak factor (trail)/9(qdz4)
  BusElementIn3/1 -> Stiffness factor (trail)/5(qbz5)
  Sum/1 -> Mz/1
  BusElementIn1/1 -> Stiffness factor (trail)/3(qbz1)
  BusElementIn10/1 -> Peak factor (trail)/8(qdz3)
  trail_slip/1 -> Aligning moment (trail)/6(trail_slip)
  Fyg0/1 -> Aligning moment (trail)/7(Fyg0)
  BusElementIn13/1 -> Peak factor (residual)/7(qdz9)
  BusElementIn15/1 -> Peak factor (residual)/9(qdz11)
  BusElementIn20/1 -> Stiffness factor (residual)/2(Cy)
  BusElementIn6/1 -> Stiffness factor (residual)/4(qbz10)
  BusElementIn9/1 -> Peak factor (trail)/7(qdz2)
  BusElementIn17/1 -> Curvature factor (trail)/7(qez2)
  BusElementIn12/1 -> Peak factor (residual)/6(qdz8)
  BusElementIn2/1 -> Stiffness factor (trail)/4(qbz2)

== system moto_linearization/moto/Subsystem/front_tire/Subsystem1/Horizontal shift ==
  dfz : Inport
  camber : Inport  Port=2
  BusElementIn : Inport  Port=3  PortName=MF  Element=qhz3
  BusElementIn1 : Inport  Port=3  PortName=MF  Element=qhz4
  Product : Product
  Product1 : Product
  Sum : Sum  Inputs=|++
  SHr : Outport
  wires:
  BusElementIn1/1 -> Product/1
  dfz/1 -> Product/2
  BusElementIn/1 -> Sum/1
  Product/1 -> Sum/2
  Sum/1 -> Product1/1
  camber/1 -> Product1/2
  Product1/1 -> SHr/1

== system moto_linearization/moto/Subsystem/front_tire/Subsystem1/Lateral force (combined slip) ==
  Fy0 : Inport
  slip_ratio : Inport  Port=2
  slip_angle : Inport  Port=3
  BusElementIn : Inport  Port=4  PortName=MF  Element=rby1
  BusElementIn1 : Inport  Port=4  PortName=MF  Element=rby2
  BusElementIn2 : Inport  Port=4  PortName=MF  Element=rby3
  BusElementIn3 : Inport  Port=4  PortName=MF  Element=rcy1
  Combined slip : Subsystem
  Lateral stiffness factor (combined) : Subsystem
  Fy : Outport
  wires:
  Fy0/1 -> Combined slip/2(Fy0)
  Combined slip/1(Fy) -> Fy/1
  BusElementIn1/1 -> Lateral stiffness factor (combined)/3(rby2)
  BusElementIn3/1 -> Combined slip/4(Cyk)
  slip_ratio/1 -> Combined slip/3(slip_ratio)
  Lateral stiffness factor (combined)/1(Byk) -> Combined slip/1(Byk)
  slip_angle/1 -> Lateral stiffness factor (combined)/1(slip_angle)
  BusElementIn/1 -> Lateral stiffness factor (combined)/2(rby1)
  BusElementIn2/1 -> Lateral stiffness factor (combined)/4(rby3)

== system moto_linearization/moto/Subsystem/front_tire/Subsystem1/Lateral force (combined slip, no camber) ==
  Fy0 : Inport
  slip_ratio : Inport  Port=2
  slip_angle : Inport  Port=3
  BusElementIn : Inport  Port=4  PortName=MF  Element=rby1
  BusElementIn1 : Inport  Port=4  PortName=MF  Element=rby2
  BusElementIn2 : Inport  Port=4  PortName=MF  Element=rby3
  BusElementIn3 : Inport  Port=4  PortName=MF  Element=rcy1
  Combined slip : Subsystem
  Lateral stiffness factor (combined) : Subsystem
  Fy : Outport
  wires:
  Fy0/1 -> Combined slip/2(Fy0)
  Combined slip/1(Fy) -> Fy/1
  BusElementIn1/1 -> Lateral stiffness factor (combined)/3(rby2)
  BusElementIn3/1 -> Combined slip/4(Cyk)
  slip_ratio/1 -> Combined slip/3(slip_ratio)
  Lateral stiffness factor (combined)/1(Byk) -> Combined slip/1(Byk)
  slip_angle/1 -> Lateral stiffness factor (combined)/1(slip_angle)
  BusElementIn/1 -> Lateral stiffness factor (combined)/2(rby1)
  BusElementIn2/1 -> Lateral stiffness factor (combined)/4(rby3)

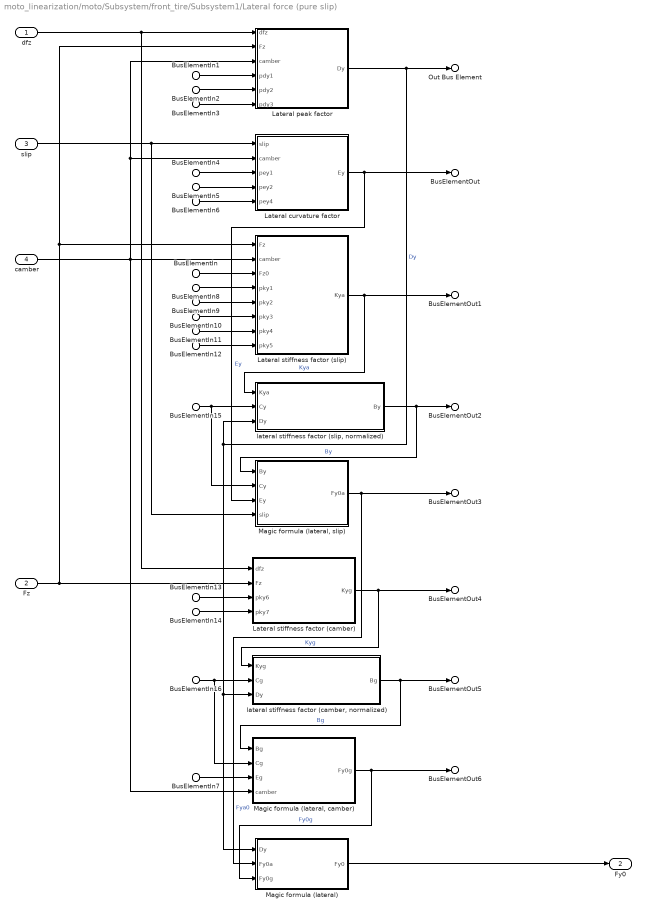
== system moto_linearization/moto/Subsystem/front_tire/Subsystem1/Lateral force (pure slip) ==
  dfz : Inport
  Fz : Inport  Port=2
  slip : Inport  Port=3
  camber : Inport  Port=4
  BusElementIn : Inport  Port=5  PortName=MF  Element=fz0
  BusElementIn1 : Inport  Port=5  PortName=MF  Element=pdy1
  BusElementIn2 : Inport  Port=5  PortName=MF  Element=pdy2
  BusElementIn3 : Inport  Port=5  PortName=MF  Element=pdy3
  BusElementIn4 : Inport  Port=5  PortName=MF  Element=pey1
  BusElementIn5 : Inport  Port=5  PortName=MF  Element=pey2
  BusElementIn6 : Inport  Port=5  PortName=MF  Element=pey4
  BusElementIn7 : Inport  Port=5  PortName=MF  Element=pey5
  BusElementIn8 : Inport  Port=5  PortName=MF  Element=pky1
  BusElementIn9 : Inport  Port=5  PortName=MF  Element=pky2
  BusElementIn10 : Inport  Port=5  PortName=MF  Element=pky3
  BusElementIn11 : Inport  Port=5  PortName=MF  Element=pky4
  BusElementIn12 : Inport  Port=5  PortName=MF  Element=pky5
  BusElementIn13 : Inport  Port=5  PortName=MF  Element=pky6
  BusElementIn14 : Inport  Port=5  PortName=MF  Element=pky7
  BusElementIn15 : Inport  Port=5  PortName=MF  Element=pcy1
  BusElementIn16 : Inport  Port=5  PortName=MF  Element=pcy2
  Lateral curvature factor : Subsystem
  Lateral peak factor : Subsystem
  Lateral stiffness factor (camber) : Subsystem
  Lateral stiffness factor (slip) : Subsystem
  Magic formula (lateral) : Subsystem
  "Magic formula (lateral, camber)" : Subsystem
  "Magic formula (lateral, slip)" : Subsystem
  "lateral stiffness factor (camber, normalized)" : Subsystem
  "lateral stiffness factor (slip, normalized)" : Subsystem
  Out Bus Element : Outport  PortName=Info  Element=Dy
  BusElementOut : Outport  PortName=Info  Element=Ey
  BusElementOut1 : Outport  PortName=Info  Element=Kya
  BusElementOut2 : Outport  PortName=Info  Element=By
  BusElementOut3 : Outport  PortName=Info  Element=Fy0a
  BusElementOut4 : Outport  PortName=Info  Element=Kyg
  BusElementOut5 : Outport  PortName=Info  Element=Bg
  BusElementOut6 : Outport  PortName=Info  Element=Fy0g
  Fy0 : Outport  Port=2
  wires:
  "Magic formula (lateral, slip)"/1(Fy0a) -> BusElementOut3/1, Magic formula (lateral)/2(Fy0a)  "Fya0"
  "Magic formula (lateral, camber)"/1(Fy0g) -> BusElementOut6/1, Magic formula (lateral)/3(Fy0g)  "Fy0g"
  dfz/1 -> Lateral peak factor/1(dfz), Lateral stiffness factor (camber)/1(dfz)
  BusElementIn/1 -> Lateral stiffness factor (slip)/3(Fz0)
  Fz/1 -> Lateral peak factor/2(Fz), Lateral stiffness factor (slip)/1(Fz), Lateral stiffness factor (camber)/2(Fz)
  BusElementIn3/1 -> Lateral peak factor/6(pdy3)
  BusElementIn12/1 -> Lateral stiffness factor (slip)/8(pky5)
  BusElementIn14/1 -> Lateral stiffness factor (camber)/4(pky7)
  Lateral stiffness factor (camber)/1(Kyg) -> BusElementOut4/1, "lateral stiffness factor (camber, normalized)"/1(Kyg)  "Kyg"
  camber/1 -> "Magic formula (lateral, camber)"/4(camber), Lateral stiffness factor (slip)/2(camber), Lateral peak factor/3(camber), Lateral curvature factor/2(camber)
  "lateral stiffness factor (camber, normalized)"/1(Bg) -> BusElementOut5/1, "Magic formula (lateral, camber)"/1(Bg)  "Bg"
  BusElementIn9/1 -> Lateral stiffness factor (slip)/5(pky2)
  Magic formula (lateral)/1(Fy0) -> Fy0/1
  BusElementIn13/1 -> Lateral stiffness factor (camber)/3(pky6)
  BusElementIn11/1 -> Lateral stiffness factor (slip)/7(pky4)
  BusElementIn15/1 -> "Magic formula (lateral, slip)"/2(Cy), "lateral stiffness factor (slip, normalized)"/2(Cy)
  BusElementIn8/1 -> Lateral stiffness factor (slip)/4(pky1)
  BusElementIn10/1 -> Lateral stiffness factor (slip)/6(pky3)
  BusElementIn4/1 -> Lateral curvature factor/3(pey1)
  slip/1 -> Lateral curvature factor/1(slip), "Magic formula (lateral, slip)"/4(slip)
  BusElementIn6/1 -> Lateral curvature factor/5(pey4)
  BusElementIn16/1 -> "Magic formula (lateral, camber)"/2(Cg), "lateral stiffness factor (camber, normalized)"/2(Cg)
  BusElementIn7/1 -> "Magic formula (lateral, camber)"/3(Eg)
  BusElementIn5/1 -> Lateral curvature factor/4(pey2)
  Lateral peak factor/1(Dy) -> Magic formula (lateral)/1(Dy), "lateral stiffness factor (camber, normalized)"/3(Dy), "lateral stiffness factor (slip, normalized)"/3(Dy), Out Bus Element/1  "Dy"
  "lateral stiffness factor (slip, normalized)"/1(By) -> BusElementOut2/1, "Magic formula (lateral, slip)"/1(By)  "By"
  Lateral stiffness factor (slip)/1(Kya) -> BusElementOut1/1, "lateral stiffness factor (slip, normalized)"/1(Kya)  "Kya"
  BusElementIn2/1 -> Lateral peak factor/5(pdy2)
  BusElementIn1/1 -> Lateral peak factor/4(pdy1)
  Lateral curvature factor/1(Ey) -> BusElementOut/1, "Magic formula (lateral, slip)"/3(Ey)  "Ey"
